simulink model "scheme"  (R2016b)
settings: Solver=VariableStepAuto  StartTime=0.0  StopTime=2  MaxStep=0.01  RelTol=1e-4  EnableMultiTasking=on
settings Model: Creator=wildm  LastModifiedBy=wildm
settings DataIOCC: LimitDataPoints=on  SaveOutput=off  SaveTime=off
settings OptimizationCC: ExpressionDepthLimit=2147483647  LifeSpan=1
settings DebuggingCC: UnderspecifiedInitializationDetection=Classic  MergeDetectMultiDrivingBlocksExec=none  FcnCallInpInsideContextMsg=warning  AllowSymbolicDim=off  StateNameClashWarn=warning  SFUnexpectedBacktrackingDiag=warning  SFNoUnconditionalDefaultTransitionDiag=warning  SFExecutionAtInitializationDiag=none
settings GRTTargetCC: TargetLangStandard=C89/C90 (ANSI)  GeneratePreprocessorConditionals=Disable all  CombineOutputUpdateFcns=off  GRTInterface=on

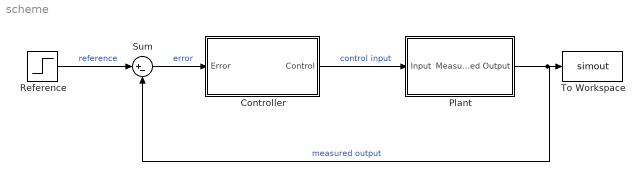
== system scheme ==
  Controller : Subsystem
  Plant : Subsystem
  Reference : Step  SampleTime=0
  Sum : Sum  Inputs=|+-
  To Workspace : ToWorkspace  VariableName=simout  SaveFormat=Timeseries  SampleTime=-1
  wires:
  Reference/1 -> Sum/1  "reference"
  Plant/1(Measured Output) -> To Workspace/1, Sum/2  "measured output"
  Sum/1 -> Controller/1(Error)  "error"
  Controller/1(Control) -> Plant/1(Input)  "control input"

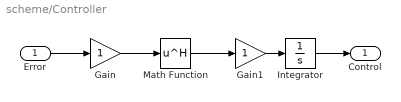
== system scheme/Controller ==
  Error : Inport
  Gain : Gain
  Gain1 : Gain
  Integrator : Integrator
  Math Function : Math  Operator=hermitian  SaturateOnIntegerOverflow=on
  Control : Outport
  wires:
  Error/1 -> Gain/1
  Math Function/1 -> Gain1/1
  Gain/1 -> Math Function/1
  Integrator/1 -> Control/1
  Gain1/1 -> Integrator/1

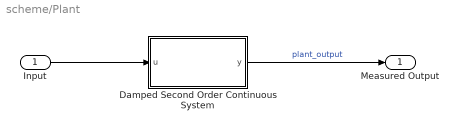
== system scheme/Plant ==
  Input : Inport
  Damped Second Order Continuous System : Subsystem  mask{wn=16, zeta=0.6}
      mask prompts: wn "Undamped natural frequency (wn, rad/s)"; zeta "Damping factor (zeta)"
  Measured Output : Outport
  wires:
  Input/1 -> Damped Second Order Continuous System/1(u)
  Damped Second Order Continuous System/1(y) -> Measured Output/1  "plant_output"

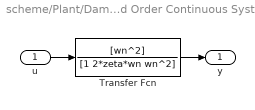
== system scheme/Plant/Damped Second Order Continuous System ==
  u : Inport
  Transfer Fcn : TransferFcn  Numerator=[wn^2]  Denominator=[1 2*zeta*wn wn^2]
  y : Outport
  wires:
  Transfer Fcn/1 -> y/1
  u/1 -> Transfer Fcn/1
